simulink model "controllo_simulink"  (R2024b)
settings: Solver=VariableStepAuto  StartTime=0.0  StopTime=20  RelTol=1e-3
values from neighbouring files (symbols this model uses):
  A = 4.8    [pw_4.mat]
undefined symbols (not defined in the file or in its folder): B, G_z, H_z, pw_2_media, R_z
settings Model: Creator=emili  LastModifiedBy=emili

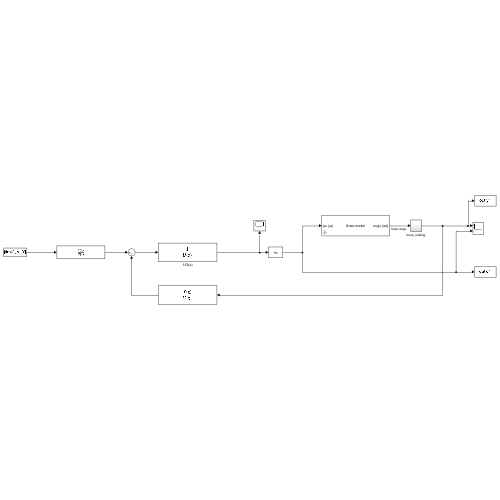
[thumbnail: Simulink's stored preview of the top-level diagram]
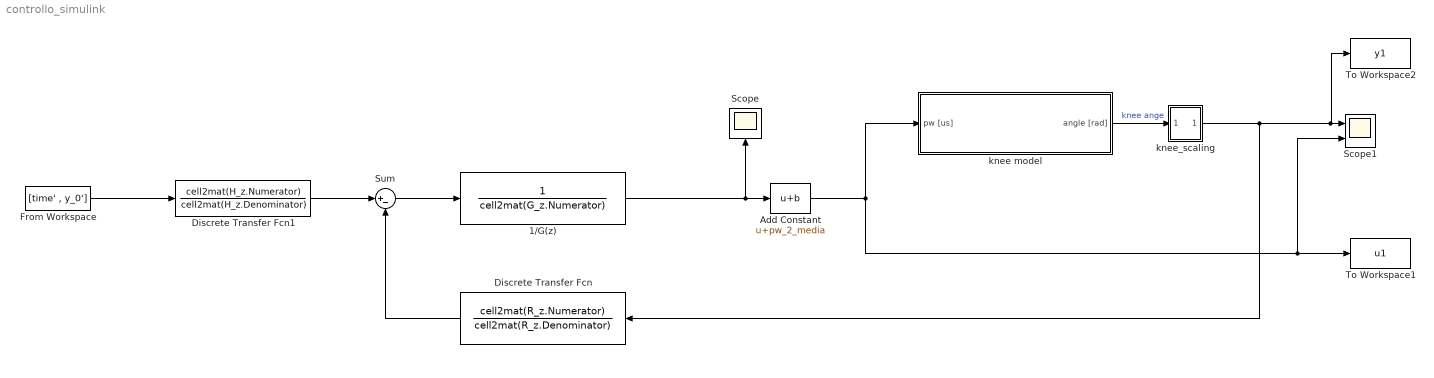
== system controllo_simulink ==
  1/G(z) : DiscreteTransferFcn  Numerator=1  Denominator=cell2mat(G_z.Numerator)
  Add Constant : Bias  Bias=pw_2_media  SaturateOnIntegerOverflow=off
  Discrete Transfer Fcn : DiscreteTransferFcn  Numerator=cell2mat(R_z.Numerator)  Denominator=cell2mat(R_z.Denominator)
  Discrete Transfer Fcn1 : DiscreteTransferFcn  Numerator=cell2mat(H_z.Numerator)  Denominator=cell2mat(H_z.Denominator)
  From Workspace : FromWorkspace  VariableName=[time' , y_0']
  Scope : Scope
  Scope1 : Scope  NumInputPorts=2
  Sum : Sum  Inputs=|+-
  To Workspace1 : ToWorkspace  VariableName=u1  SampleTime=0.05
  To Workspace2 : ToWorkspace  VariableName=y1  SampleTime=0.05
  knee model : Subsystem  mask{freq=20, qk0=1.54248, act0=[0 0 0 0 0 0    0 0 0.0 0 0.0 0   0 0 0 0 0 0 ]}
      mask prompts: freq "frequency:"; qk0 "initial knee angle:"; act0 "initial states for musle activation:"
      mask init:
      | [A,B]=creAB;
      mask Display: disp('Knee model')
  knee_scaling : Subsystem
  wires:
  Sum/1 -> 1/G(z)/1
  Discrete Transfer Fcn/1 -> Sum/2
  Discrete Transfer Fcn1/1 -> Sum/1
  knee model/1(angle [rad]) -> knee_scaling/1(in_1)  "knee ange"
  knee_scaling/1(knee_angle_[deg]) -> Discrete Transfer Fcn/1, To Workspace2/1, Scope1/1
  From Workspace/1 -> Discrete Transfer Fcn1/1
  1/G(z)/1 -> Add Constant/1, Scope/1
  Add Constant/1 -> knee model/1(pw [us]), Scope1/2, To Workspace1/1

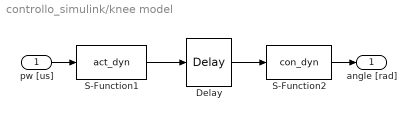
== system controllo_simulink/knee model ==
  pw [us] : Inport
  Delay : TransportDelay  DelayTime=0.025  InitialOutput=act0(1:2:17)
  S-Function1 : S-Function  FunctionName=act_dyn  Parameters=act0,freq,A,B  SFunctionDeploymentMode=off  EnableBusSupport=off
  S-Function2 : S-Function  FunctionName=con_dyn  Parameters=qk0  SFunctionDeploymentMode=off  EnableBusSupport=off
  angle [rad] : Outport  InitialOutput=0
  wires:
  S-Function1/1 -> Delay/1
  pw [us]/1 -> S-Function1/1
  S-Function2/1 -> angle [rad]/1
  Delay/1 -> S-Function2/1

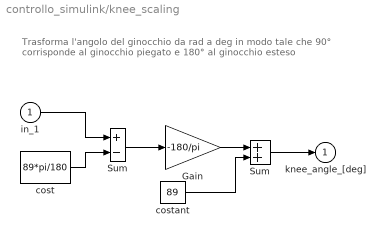
== system controllo_simulink/knee_scaling ==
  note: Trasforma l'angolo del ginocchio da rad a deg in modo tale che
      | 90° corrisponde al ginocchio piegato e 180° al ginocchio esteso
  in_1 : Inport
  Gain : Gain  Gain=-180/pi  SaturateOnIntegerOverflow=on  OutDataTypeStr=Inherit: Same as input  ParamDataTypeStr=Inherit: Same as input
  "Sum " : Sum  Inputs=+-  InputSameDT=on  SaturateOnIntegerOverflow=on  OutDataTypeStr=Inherit: Same as first input
  "Sum " : Sum  InputSameDT=on  SaturateOnIntegerOverflow=on  OutDataTypeStr=Inherit: Same as first input
  cost : Constant  Value=89*pi/180
  "costant " : Constant  Value=89
  knee_angle_[deg] : Outport  InitialOutput=0
  wires:
  "Sum "/1 -> knee_angle_[deg]/1
  in_1/1 -> "Sum "/1
  cost/1 -> "Sum "/2
  "Sum "/1 -> Gain/1
  Gain/1 -> "Sum "/1
  "costant "/1 -> "Sum "/2
